simulink model "AtmLast2Real"  (R2015a)
settings: configuration reference "SIMULATION_CONFIGURATION" (kept outside this file)
settings Model: CovSFcnEnable=off  Creator=moritz  LastModifiedBy=moritz
settings ConfigSetRef: SourceLocation=Base Workspace

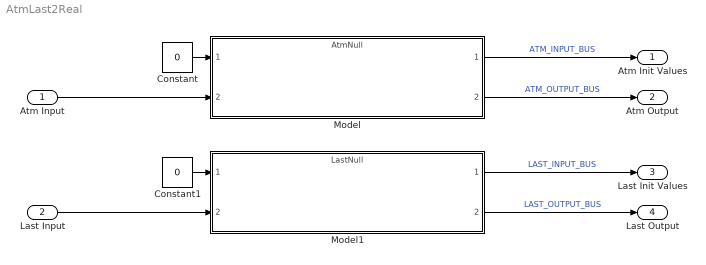
== system AtmLast2Real ==
  Atm Input : Inport  OutDataTypeStr=Bus: ATM_INPUT_BUS  BusOutputAsStruct=on
  Last Input : Inport  Port=2  OutDataTypeStr=Bus: LAST_INPUT_BUS  BusOutputAsStruct=on
  Constant : Constant  Value=0  OutDataTypeStr=boolean
  Constant1 : Constant  Value=0  OutDataTypeStr=boolean
  Model : ModelReference  ModelNameDialog=AtmNull  Variant=on  ModelReferenceVersion=1.19  CopyOfModelName=AtmNull  DefaultDataLogging=on
  Model1 : ModelReference  ModelNameDialog=LastNull  Variant=on  ModelReferenceVersion=1.22  CopyOfModelName=LastNull  DefaultDataLogging=on
  Atm Init Values : Outport  OutDataTypeStr=Bus: ATM_INPUT_BUS  BusOutputAsStruct=on
  Atm Output : Outport  Port=2  OutDataTypeStr=Bus: ATM_OUTPUT_BUS  BusOutputAsStruct=on
  Last Init Values : Outport  Port=3  OutDataTypeStr=Bus: LAST_OUTPUT_BUS  BusOutputAsStruct=on
  Last Output : Outport  Port=4  OutDataTypeStr=Bus: LAST_INPUT_BUS  BusOutputAsStruct=on
  wires:
  Model/1 -> Atm Init Values/1  "ATM_INPUT_BUS"
  Model1/1 -> Last Init Values/1  "LAST_INPUT_BUS"
  Model/2 -> Atm Output/1  "ATM_OUTPUT_BUS"
  Model1/2 -> Last Output/1  "LAST_OUTPUT_BUS"
  Atm Input/1 -> Model/2
  Last Input/1 -> Model1/2
  Constant/1 -> Model/1
  Constant1/1 -> Model1/1
